simulink model "lab2q3blockdiagram"  (Simulink 8.7)
settings: Solver=VariableStepAuto  StartTime=0.0  StopTime=3  RelTol=1e-3
settings Model: Creator=gmcma  LastModifiedBy=gmcma
settings DataIOCC: LimitDataPoints=off  SaveFormat=Dataset
settings DebuggingCC: UnderspecifiedInitializationDetection=Simplified  MergeDetectMultiDrivingBlocksExec=error
settings HardwareCC: ProdBitPerPointer=64  ProdLargestAtomicFloat=Float  ProdIntDivRoundTo=Zero  ProdEndianess=LittleEndian  ProdWordSize=64  ProdHWDeviceType=Intel->x86-64 (Windows64)
settings ModelReferenceCC: PropagateSignalLabelsOutOfModel=on
settings ConfigComp: CovModelRefEnable=off

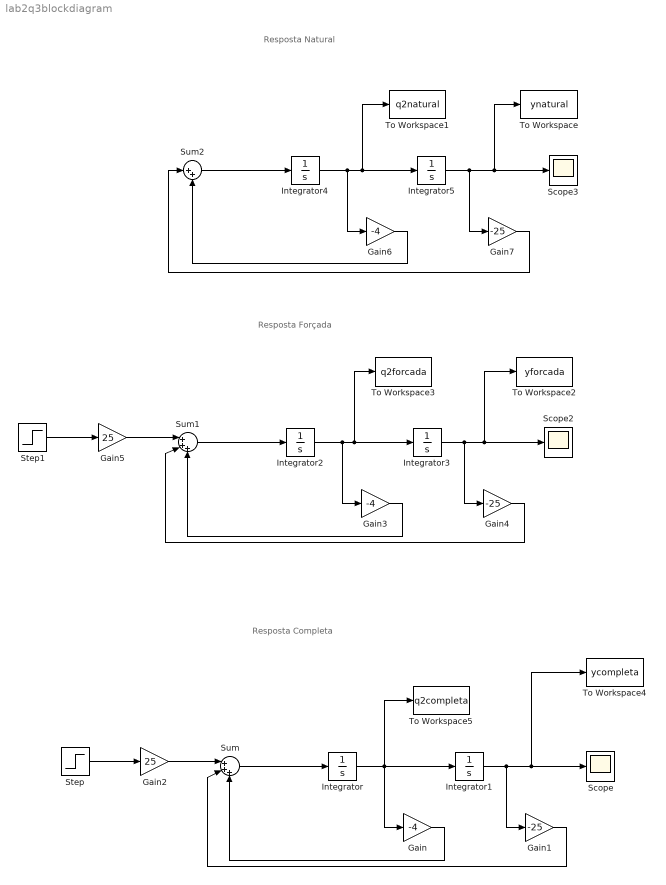
== system lab2q3blockdiagram ==
  note: Resposta Completa
  note: Resposta Natural
  note: Resposta Forçada
  Gain : Gain  Gain=-4
  Gain1 : Gain  Gain=-25
  Gain2 : Gain  Gain=25
  Gain3 : Gain  Gain=-4
  Gain4 : Gain  Gain=-25
  Gain5 : Gain  Gain=25
  Gain6 : Gain  Gain=-4
  Gain7 : Gain  Gain=-25
  Integrator : Integrator  InitialCondition=3
  Integrator1 : Integrator  InitialCondition=1
  Integrator2 : Integrator
  Integrator3 : Integrator
  Integrator4 : Integrator  InitialCondition=3
  Integrator5 : Integrator  InitialCondition=1
  Scope : Scope
  Scope2 : Scope
  Scope3 : Scope
  Step : Step  Time=0  SampleTime=0
  Step1 : Step  Time=0  SampleTime=0
  Sum : Sum  Inputs=|+++
  Sum1 : Sum  Inputs=|+++
  Sum2 : Sum  Inputs=|++
  To Workspace : ToWorkspace  VariableName=ynatural  SaveFormat=Structure With Time  SampleTime=-1
  To Workspace1 : ToWorkspace  VariableName=q2natural  SaveFormat=Structure With Time  SampleTime=-1
  To Workspace2 : ToWorkspace  VariableName=yforcada  SaveFormat=Structure With Time  SampleTime=-1
  To Workspace3 : ToWorkspace  VariableName=q2forcada  SaveFormat=Structure With Time  SampleTime=-1
  To Workspace4 : ToWorkspace  VariableName=ycompleta  SaveFormat=Structure With Time  SampleTime=-1
  To Workspace5 : ToWorkspace  VariableName=q2completa  SaveFormat=Structure With Time  SampleTime=-1
  wires:
  Step/1 -> Gain2/1
  Gain2/1 -> Sum/1
  Sum/1 -> Integrator/1
  Integrator/1 -> To Workspace5/1, Gain/1, Integrator1/1
  Integrator1/1 -> To Workspace4/1, Scope/1, Gain1/1
  Gain1/1 -> Sum/2
  Gain/1 -> Sum/3
  Step1/1 -> Gain5/1
  Gain5/1 -> Sum1/1
  Sum1/1 -> Integrator2/1
  Integrator2/1 -> Gain3/1, To Workspace3/1, Integrator3/1
  Integrator3/1 -> To Workspace2/1, Scope2/1, Gain4/1
  Gain4/1 -> Sum1/2
  Gain3/1 -> Sum1/3
  Sum2/1 -> Integrator4/1
  Gain6/1 -> Sum2/2
  Gain7/1 -> Sum2/1
  Integrator5/1 -> To Workspace/1, Scope3/1, Gain7/1
  Integrator4/1 -> Gain6/1, To Workspace1/1, Integrator5/1
